simulink model "Get_SEPs"  (R2013b)
settings: Solver=ode45  StartTime=0.0  StopTime=Inf  RelTol=1e-3
undefined symbols (not defined in the file or in its folder): currentCFG_Get_SEPs_UB, UB
libraries: gUSBamplib x2
settings Model: Creator=JaimeIbanez  LastModifiedBy=FranR

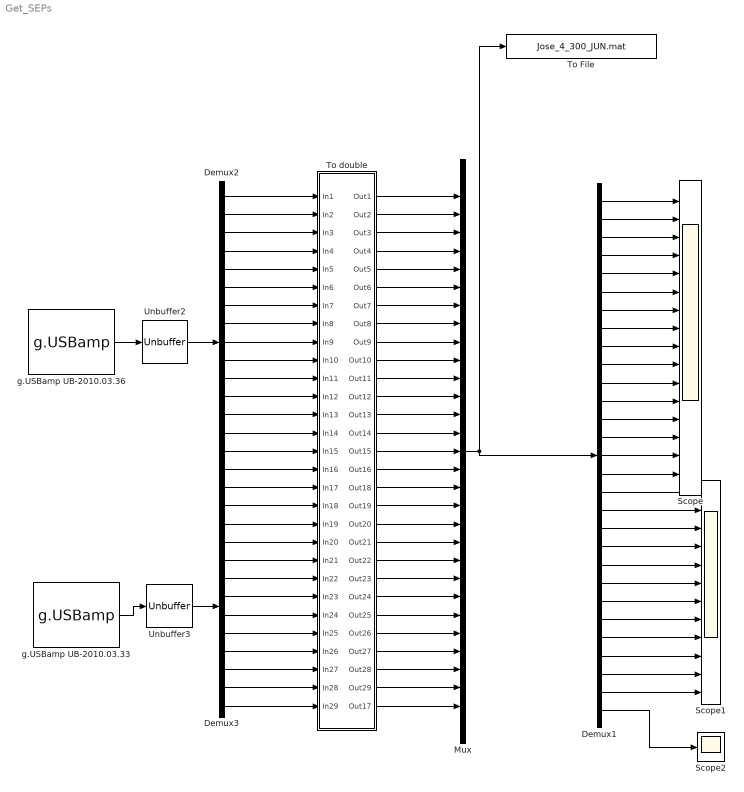
== system Get_SEPs ==
  Demux1 : Demux  Outputs=29
  Demux2 : Demux  Outputs=17
  Demux3 : Demux  Outputs=12
  Mux : Mux  Inputs=29
  Scope : Scope  NumInputPorts=16
      settings: TickLabels=off  TimeRange=10  YMin=-5000~0~-6000~-8000~-14000~-27500~-5000~-8000~-10000~-5000~-4000~-8000~-4000~-4000~-5000~-6000  YMax=2000~9000~1000~-1000~-6000~-17500~3000~-1000~-2000~3000~4000~-1000~3000~3000~2000~1000
  Scope1 : Scope  NumInputPorts=12
      settings: TickLabels=off  TimeRange=10  YMin=-8000~-8000~2000~4000~-3500~-5000~-13000~-8000~-8500~-1500~-500~-5000  YMax=-1000~-1000~7500~9500~1500~1000~-6000~-3500~-4000~3000~4000~0
  Scope2 : Scope
      settings: SaveName=ScopeData2
  To File : ToFile  Filename=Jose_4_300_JUN.mat  MatrixName=data
  To double : Subsystem
  Unbuffer2 : Unbuffer
  Unbuffer3 : Unbuffer
  g.USBamp UB-2010.03.33 : gUSBamplib/g.USBamp  Priority=1  cfg=currentCFG_Get_SEPs_UB-2010.03.33.cfg  snr=UB-2010.03.33
  g.USBamp UB-2010.03.36 : gUSBamplib/g.USBamp  Priority=2  cfg=currentCFG_Get_SEPs_UB-2010.03.36.cfg  snr=UB-2010.03.36
  wires:
  Unbuffer2/1 -> Demux2/1
  Unbuffer3/1 -> Demux3/1
  Mux/1 -> To File/1, Demux1/1
  g.USBamp UB-2010.03.33/1 -> Unbuffer3/1
  g.USBamp UB-2010.03.36/1 -> Unbuffer2/1
  To double/1(Out1) -> Mux/1
  To double/2(Out2) -> Mux/2
  To double/3(Out3) -> Mux/3
  To double/4(Out4) -> Mux/4
  To double/5(Out5) -> Mux/5
  To double/6(Out6) -> Mux/6
  To double/7(Out7) -> Mux/7
  To double/8(Out8) -> Mux/8
  To double/9(Out9) -> Mux/9
  To double/10(Out10) -> Mux/10
  To double/11(Out11) -> Mux/11
  To double/12(Out12) -> Mux/12
  To double/13(Out13) -> Mux/13
  To double/14(Out14) -> Mux/14
  To double/15(Out15) -> Mux/15
  To double/16(Out16) -> Mux/16
  To double/17(Out18) -> Mux/17
  To double/18(Out19) -> Mux/18
  To double/19(Out20) -> Mux/19
  To double/20(Out21) -> Mux/20
  To double/21(Out22) -> Mux/21
  To double/22(Out23) -> Mux/22
  To double/23(Out24) -> Mux/23
  To double/24(Out25) -> Mux/24
  To double/25(Out26) -> Mux/25
  To double/26(Out27) -> Mux/26
  To double/27(Out28) -> Mux/27
  To double/28(Out29) -> Mux/28
  To double/29(Out17) -> Mux/29
  Demux1/5 -> Scope/5
  Demux1/4 -> Scope/4
  Demux1/1 -> Scope/1
  Demux1/2 -> Scope/2
  Demux1/3 -> Scope/3
  Demux1/6 -> Scope/6
  Demux1/7 -> Scope/7
  Demux1/8 -> Scope/8
  Demux1/9 -> Scope/9
  Demux1/10 -> Scope/10
  Demux1/11 -> Scope/11
  Demux1/12 -> Scope/12
  Demux1/13 -> Scope/13
  Demux1/14 -> Scope/14
  Demux1/15 -> Scope/15
  Demux1/16 -> Scope/16
  Demux1/17 -> Scope1/1
  Demux1/18 -> Scope1/2
  Demux1/19 -> Scope1/3
  Demux1/20 -> Scope1/4
  Demux1/21 -> Scope1/5
  Demux1/22 -> Scope1/6
  Demux1/23 -> Scope1/7
  Demux1/24 -> Scope1/8
  Demux1/25 -> Scope1/9
  Demux1/26 -> Scope1/10
  Demux1/27 -> Scope1/11
  Demux1/28 -> Scope1/12
  Demux1/29 -> Scope2/1
  Demux3/1 -> To double/18(In18)
  Demux3/2 -> To double/19(In19)
  Demux3/3 -> To double/20(In20)
  Demux3/4 -> To double/21(In21)
  Demux3/5 -> To double/22(In22)
  Demux3/6 -> To double/23(In23)
  Demux3/7 -> To double/24(In24)
  Demux3/8 -> To double/25(In25)
  Demux3/9 -> To double/26(In26)
  Demux3/10 -> To double/27(In27)
  Demux3/11 -> To double/28(In28)
  Demux3/12 -> To double/29(In29)
  Demux2/1 -> To double/1(In1)
  Demux2/2 -> To double/2(In2)
  Demux2/3 -> To double/3(In3)
  Demux2/4 -> To double/4(In4)
  Demux2/5 -> To double/5(In5)
  Demux2/6 -> To double/6(In6)
  Demux2/7 -> To double/7(In7)
  Demux2/8 -> To double/8(In8)
  Demux2/9 -> To double/9(In9)
  Demux2/10 -> To double/10(In10)
  Demux2/11 -> To double/11(In11)
  Demux2/12 -> To double/12(In12)
  Demux2/13 -> To double/13(In13)
  Demux2/14 -> To double/14(In14)
  Demux2/15 -> To double/15(In15)
  Demux2/16 -> To double/16(In16)
  Demux2/17 -> To double/17(In17)

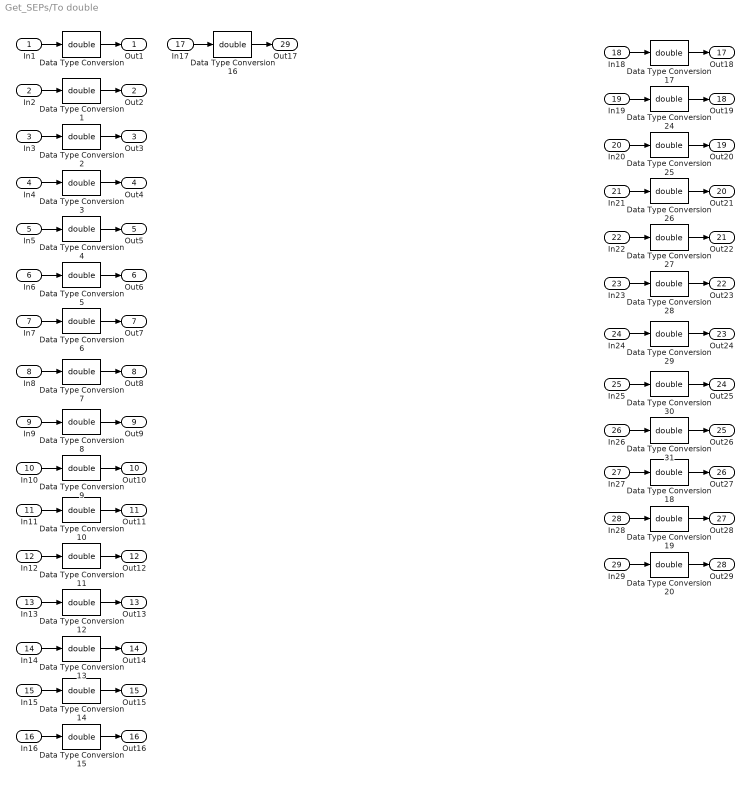
== system Get_SEPs/To double ==
  In1 : Inport
  In2 : Inport  Port=2
  In3 : Inport  Port=3
  In4 : Inport  Port=4
  In5 : Inport  Port=5
  In6 : Inport  Port=6
  In7 : Inport  Port=7
  In8 : Inport  Port=8
  In9 : Inport  Port=9
  In10 : Inport  Port=10
  In11 : Inport  Port=11
  In12 : Inport  Port=12
  In13 : Inport  Port=13
  In14 : Inport  Port=14
  In15 : Inport  Port=15
  In16 : Inport  Port=16
  In17 : Inport  Port=17
  In18 : Inport  Port=18
  In19 : Inport  Port=19
  In20 : Inport  Port=20
  In21 : Inport  Port=21
  In22 : Inport  Port=22
  In23 : Inport  Port=23
  In24 : Inport  Port=24
  In25 : Inport  Port=25
  In26 : Inport  Port=26
  In27 : Inport  Port=27
  In28 : Inport  Port=28
  In29 : Inport  Port=29
  Data Type Conversion{,1..20,24..31} (29 alike) : DataTypeConversion  OutDataTypeStr=double
  Out1 : Outport
  Out2 : Outport  Port=2
  Out3 : Outport  Port=3
  Out4 : Outport  Port=4
  Out5 : Outport  Port=5
  Out6 : Outport  Port=6
  Out7 : Outport  Port=7
  Out8 : Outport  Port=8
  Out9 : Outport  Port=9
  Out10 : Outport  Port=10
  Out11 : Outport  Port=11
  Out12 : Outport  Port=12
  Out13 : Outport  Port=13
  Out14 : Outport  Port=14
  Out15 : Outport  Port=15
  Out16 : Outport  Port=16
  Out18 : Outport  Port=17
  Out19 : Outport  Port=18
  Out20 : Outport  Port=19
  Out21 : Outport  Port=20
  Out22 : Outport  Port=21
  Out23 : Outport  Port=22
  Out24 : Outport  Port=23
  Out25 : Outport  Port=24
  Out26 : Outport  Port=25
  Out27 : Outport  Port=26
  Out28 : Outport  Port=27
  Out29 : Outport  Port=28
  Out17 : Outport  Port=29
  wires:
  In1/1 -> Data Type Conversion/1
  Data Type Conversion/1 -> Out1/1
  In2/1 -> Data Type Conversion1/1
  Data Type Conversion1/1 -> Out2/1
  In3/1 -> Data Type Conversion2/1
  Data Type Conversion2/1 -> Out3/1
  In4/1 -> Data Type Conversion3/1
  Data Type Conversion3/1 -> Out4/1
  In5/1 -> Data Type Conversion4/1
  Data Type Conversion4/1 -> Out5/1
  In6/1 -> Data Type Conversion5/1
  Data Type Conversion5/1 -> Out6/1
  In7/1 -> Data Type Conversion6/1
  Data Type Conversion6/1 -> Out7/1
  In8/1 -> Data Type Conversion7/1
  Data Type Conversion7/1 -> Out8/1
  In9/1 -> Data Type Conversion8/1
  Data Type Conversion8/1 -> Out9/1
  In10/1 -> Data Type Conversion9/1
  Data Type Conversion9/1 -> Out10/1
  In11/1 -> Data Type Conversion10/1
  Data Type Conversion10/1 -> Out11/1
  In12/1 -> Data Type Conversion11/1
  Data Type Conversion11/1 -> Out12/1
  In13/1 -> Data Type Conversion12/1
  Data Type Conversion12/1 -> Out13/1
  In14/1 -> Data Type Conversion13/1
  Data Type Conversion13/1 -> Out14/1
  In15/1 -> Data Type Conversion14/1
  Data Type Conversion14/1 -> Out15/1
  In16/1 -> Data Type Conversion15/1
  Data Type Conversion15/1 -> Out16/1
  In17/1 -> Data Type Conversion16/1
  Data Type Conversion16/1 -> Out17/1
  In18/1 -> Data Type Conversion17/1
  Data Type Conversion17/1 -> Out18/1
  In19/1 -> Data Type Conversion24/1
  Data Type Conversion24/1 -> Out19/1
  In20/1 -> Data Type Conversion25/1
  Data Type Conversion25/1 -> Out20/1
  In21/1 -> Data Type Conversion26/1
  Data Type Conversion26/1 -> Out21/1
  In22/1 -> Data Type Conversion27/1
  Data Type Conversion27/1 -> Out22/1
  In23/1 -> Data Type Conversion28/1
  Data Type Conversion28/1 -> Out23/1
  In24/1 -> Data Type Conversion29/1
  Data Type Conversion29/1 -> Out24/1
  In25/1 -> Data Type Conversion30/1
  Data Type Conversion30/1 -> Out25/1
  In26/1 -> Data Type Conversion31/1
  Data Type Conversion31/1 -> Out26/1
  In27/1 -> Data Type Conversion18/1
  Data Type Conversion18/1 -> Out27/1
  In28/1 -> Data Type Conversion19/1
  Data Type Conversion19/1 -> Out28/1
  In29/1 -> Data Type Conversion20/1
  Data Type Conversion20/1 -> Out29/1
